simulink model "lab1ex9"  (Simulink 6.0)
settings: Solver=ode45  StartTime=0.0  StopTime=10.0  RelTol=1e-3
settings Model: LastModifiedBy=student

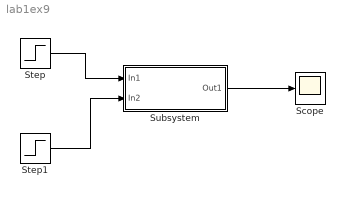
== system lab1ex9 ==
  Scope : Scope
  Step : Step  SampleTime=0
  Step1 : Step  SampleTime=0
  Subsystem : Subsystem
  wires:
  Step/1 -> Subsystem/1(In1)
  Step1/1 -> Subsystem/2(In2)
  Subsystem/1(Out1) -> Scope/1

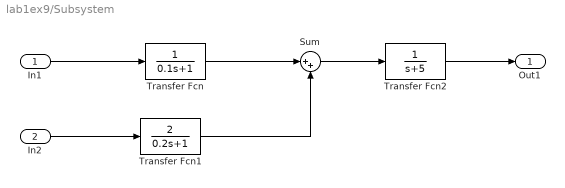
== system lab1ex9/Subsystem ==
  In1 : Inport  Port=1  LatchInput=off
  In2 : Inport  Port=2  LatchInput=off
  Sum : Sum  Inputs=|++
  Transfer Fcn : TransferFcn  Denominator=[0.1 1]
  Transfer Fcn1 : TransferFcn  Numerator=[2]  Denominator=[0.2 1]
  Transfer Fcn2 : TransferFcn  Denominator=[1 5]
  Out1 : Outport
  wires:
  Transfer Fcn/1 -> Sum/1
  In1/1 -> Transfer Fcn/1
  In2/1 -> Transfer Fcn1/1
  Transfer Fcn1/1 -> Sum/2
  Sum/1 -> Transfer Fcn2/1
  Transfer Fcn2/1 -> Out1/1
